simulink model "model_cessna182_long"  (R2013a)
settings: Solver=ode45  StartTime=0.0  StopTime=200  MaxStep=0.01  RelTol=1e-3
InitFcn:
  | cessna182
values from neighbouring files (symbols this model uses):
  Clong = eye(4)    [cessna182.m]
  Dlong = zeros (4,1)    [cessna182.m]
  Kc = 0.0741    [cessna182_long.m]
undefined symbols (not defined in the file or in its folder): Along, Blong
settings Model: Creator=Aluno  LastModifiedBy=Aluno

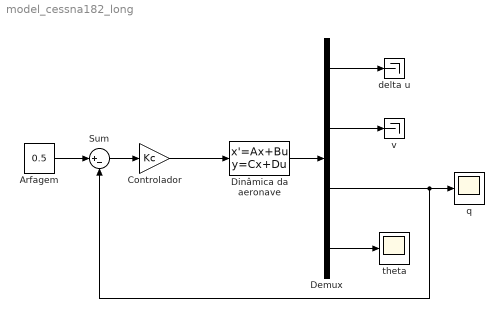
== system model_cessna182_long ==
  Arfagem : Constant  Value=0.5
  Controlador : Gain  Gain=Kc
  Demux : Demux
  Dinâmica da aeronave : StateSpace  A=Along  B=Blong  C=Clong  D=Dlong
  Sum : Sum  Inputs=|+-
  delta u : Terminator
  q : Scope
      settings: SaveName=q
  theta : Scope
      settings: SaveName=theta
  v : Terminator
  wires:
  Arfagem/1 -> Sum/1
  Sum/1 -> Controlador/1
  Controlador/1 -> Dinâmica da aeronave/1
  Dinâmica da aeronave/1 -> Demux/1
  Demux/3 -> q/1, Sum/2
  Demux/2 -> v/1
  Demux/1 -> delta u/1
  Demux/4 -> theta/1
